simulink model "simu7"  (R2018a)
settings: Solver=VariableStepAuto  StartTime=0.0  StopTime=10.0  RelTol=1e-3
values from neighbouring files (symbols this model uses):
  T = 0.5    [TimeResponseof1stn2ndorder.m]    (also in pgo7.m)
libraries: simulink x1
settings Model: Creator=SHRUTI  LastModifiedBy=SHRUTI

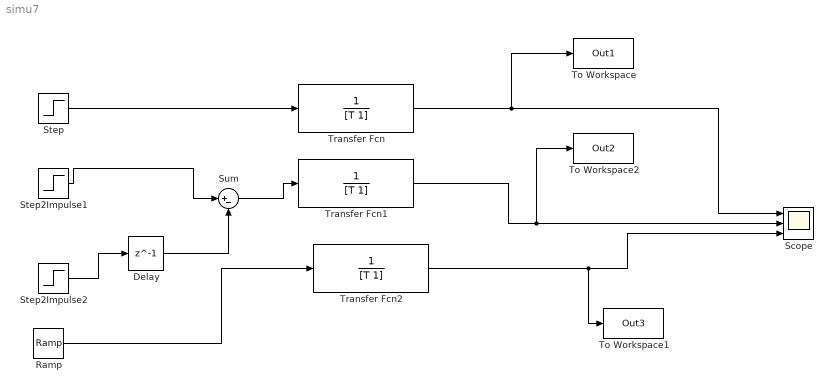
== system simu7 ==
  Delay : Delay  DelayLength=1
  Ramp : simulink/Sources/Ramp  slope=1  start=0  InitialOutput=0
  Scope : Scope  NumInputPorts=3
  Step : Step  Time=0  SampleTime=0
  Step2Impulse1 : Step  Time=0  SampleTime=0
  Step2Impulse2 : Step  Time=0  SampleTime=0
  Sum : Sum  Inputs=|+-
  To Workspace : ToWorkspace  VariableName=Out1  SampleTime=-1
  To Workspace1 : ToWorkspace  VariableName=Out3  SampleTime=-1
  To Workspace2 : ToWorkspace  VariableName=Out2  SampleTime=-1
  Transfer Fcn : TransferFcn  Denominator=[T 1]
  Transfer Fcn1 : TransferFcn  Denominator=[T 1]
  Transfer Fcn2 : TransferFcn  Denominator=[T 1]
  wires:
  Step2Impulse2/1 -> Delay/1
  Delay/1 -> Sum/2
  Step2Impulse1/1 -> Sum/1
  Step/1 -> Transfer Fcn/1
  Sum/1 -> Transfer Fcn1/1
  Ramp/1 -> Transfer Fcn2/1
  Transfer Fcn/1 -> To Workspace/1, Scope/1
  Transfer Fcn1/1 -> To Workspace2/1, Scope/2
  Transfer Fcn2/1 -> To Workspace1/1, Scope/3
